simulink model "stableMDS_variable_stiffness"  (R2020b)
settings: Solver=FixedStepAuto  StartTime=0.0  StopTime=10.0  FixedStep=0.001  RelTol=1e-3
values from neighbouring files (symbols this model uses):
  a0 = 0.99    [init.m]
  berta = 0.98    [init.m]
  csi = 1    [init.m]
  e_max = 0.05    [init.m]
  F_max = [2;2]    [init.m]
  F_weight = [0;-50]    [init.m]
  M = 1    [init.m]
  mass = 1    [init.m]
libraries: cstblocks x2
settings Model: Creator=chiara-s  LastModifiedBy=chiara-s

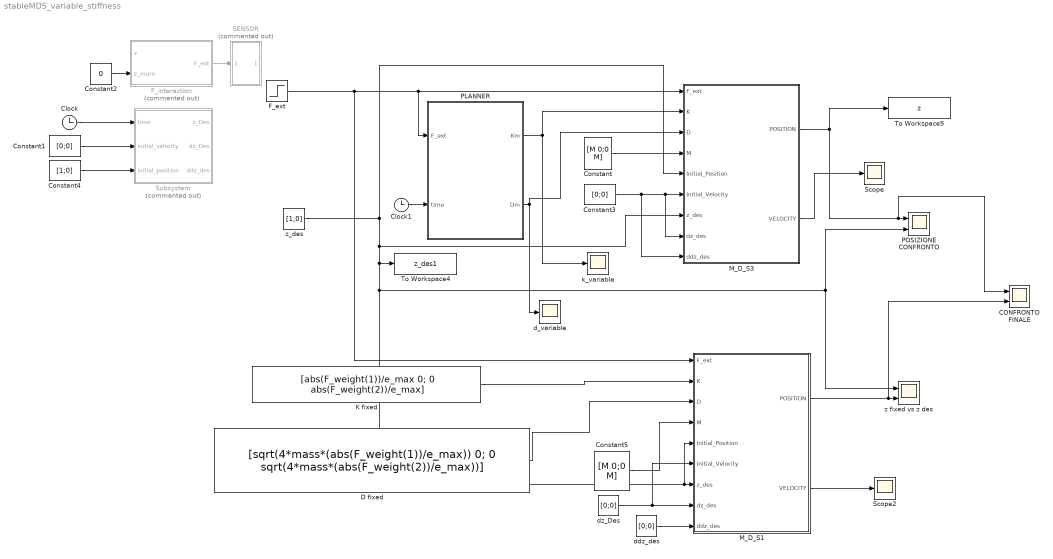
== system stableMDS_variable_stiffness ==
  CONFRONTO FINALE : Scope  NumInputPorts=2
  Clock : Clock
  Clock1 : Clock
  Constant : Constant  Value=[M 0;0 M]
  Constant1 : Constant  Value=[0;0]
  Constant2 : Constant  Value=0
  Constant3 : Constant  Value=[0;0]
  Constant4 : Constant  Value=[1;0]
  Constant5 : Constant  Value=[M 0;0 M]
  D fixed : Constant  Value=[sqrt(4*mass*(abs(F_weight(1))/e_max)) 0; 0 sqrt(4*mass*(abs(F_weight(2))/e_max))]
  F_ext : Step  Before=[0;0]  After=2*F_weight  SampleTime=0
  F_interaction : MATLAB Function  Commented=on  TreatAsAtomicUnit=on
  K fixed : Constant  Value=[abs(F_weight(1))/e_max 0; 0 abs(F_weight(2))/e_max]
  M_D_S1 : Subsystem
  M_D_S3 : Subsystem
  PLANNER : MATLAB Function  TreatAsAtomicUnit=on
  POSIZIONE CONFRONTO : Scope  NumInputPorts=2
  SENSOR : Subsystem  Commented=on
  Scope : Scope
  Scope2 : Scope
  Subsystem : Subsystem  Commented=on
  To Workspace4 : ToWorkspace  VariableName=z_des1  SaveFormat=Structure With Time  SampleTime=-1
      settings: Save2DSignal=2-D array (concatenate along first dimension)
  To Workspace5 : ToWorkspace  VariableName=z  SaveFormat=Structure With Time  SampleTime=-1
  d_variable : Scope
  ddz_des : Constant  Value=[0;0]
  dz_Des : Constant  Value=[0;0]
  k_variable : Scope
  z fixed vs z des : Scope  NumInputPorts=2
  z_des : Constant  Value=[1;0]
  wires:
  M_D_S3/2(VELOCITY) -> Scope/1
  ddz_des/1 -> M_D_S1/9(ddz_des)
  dz_Des/1 -> M_D_S1/8(dz_des), M_D_S1/6(Initial_Velocity)
  Constant4/1 -> Subsystem/3(initial_position)
  Constant1/1 -> Subsystem/2(initial_velocity)
  z_des/1 -> M_D_S3/5(Initial_Position), M_D_S1/5(Initial_Position), M_D_S1/7(z_des), z fixed vs z des/1, POSIZIONE CONFRONTO/2, To Workspace4/1, M_D_S3/7(z_des)
  PLANNER/1(Km) -> k_variable/1, M_D_S3/2(K)
  M_D_S3/1(POSITION) -> To Workspace5/1, CONFRONTO FINALE/1, POSIZIONE CONFRONTO/1
  F_interaction/1(F_ext) -> SENSOR/1(In1)
  Constant2/1 -> F_interaction/2(z_muro)
  D fixed/1 -> M_D_S1/3(D)
  Constant/1 -> M_D_S3/4(M)
  PLANNER/2(Dm) -> M_D_S3/3(D), d_variable/1
  K fixed/1 -> M_D_S1/2(K)
  Clock/1 -> Subsystem/1(time)
  Constant3/1 -> M_D_S3/6(Initial_Velocity), M_D_S3/8(dz_des), M_D_S3/9(ddz_des)
  M_D_S1/2(VELOCITY) -> Scope2/1
  Constant5/1 -> M_D_S1/4(M)
  M_D_S1/1(POSITION) -> CONFRONTO FINALE/2, z fixed vs z des/2
  Clock1/1 -> PLANNER/2(time)
  F_ext/1 -> PLANNER/1(F_ext), M_D_S3/1(F_ext), M_D_S1/1(F_ext)

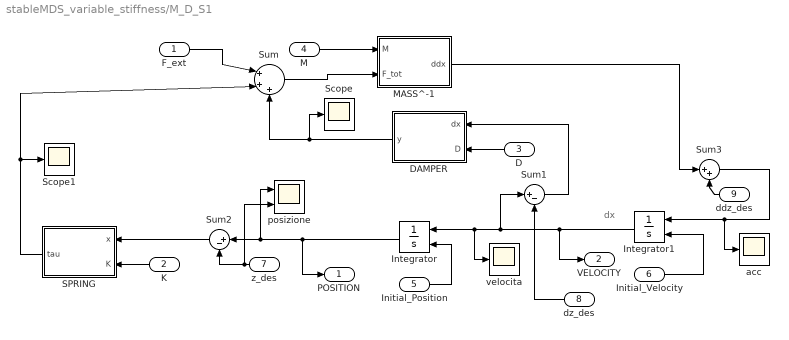
== system stableMDS_variable_stiffness/M_D_S1 ==
  note: dx
  F_ext : Inport
  K : Inport  Port=2
  D : Inport  Port=3
  M : Inport  Port=4
  Initial_Position : Inport  Port=5
  Initial_Velocity : Inport  Port=6
  z_des : Inport  Port=7
  dz_des : Inport  Port=8
  ddz_des : Inport  Port=9
  DAMPER : MATLAB Function  TreatAsAtomicUnit=on
  Integrator : Integrator  InitialConditionSource=external
  Integrator1 : Integrator  InitialConditionSource=external
  MASS^-1 : MATLAB Function  TreatAsAtomicUnit=on
  SPRING : MATLAB Function  TreatAsAtomicUnit=on
  Scope : Scope
  Scope1 : Scope
  Sum : Sum  Inputs=|+++
  Sum1 : Sum  Inputs=|+-
  Sum2 : Sum  Inputs=|+-
  Sum3 : Sum  Inputs=|++
  acc : Scope
  posizione : Scope  NumInputPorts=2
  velocita : Scope
  POSITION : Outport
  VELOCITY : Outport  Port=2
  wires:
  Integrator1/1 -> velocita/1, Integrator/1, Sum1/1, VELOCITY/1
  SPRING/1(tau) -> Sum/2, Scope1/1
  Integrator/1 -> posizione/1, Sum2/1, POSITION/1
  DAMPER/1(y) -> Scope/1, Sum/3
  Sum/1 -> MASS^-1/2(F_tot)
  M/1 -> MASS^-1/1(M)
  D/1 -> DAMPER/2(D)
  K/1 -> SPRING/2(K)
  Initial_Velocity/1 -> Integrator1/2
  Initial_Position/1 -> Integrator/2
  z_des/1 -> posizione/2, Sum2/2
  Sum2/1 -> SPRING/1(x)
  MASS^-1/1(ddx) -> Sum3/1
  Sum1/1 -> DAMPER/1(dx)
  Sum3/1 -> acc/1, Integrator1/1
  dz_des/1 -> Sum1/2
  ddz_des/1 -> Sum3/2
  F_ext/1 -> Sum/1

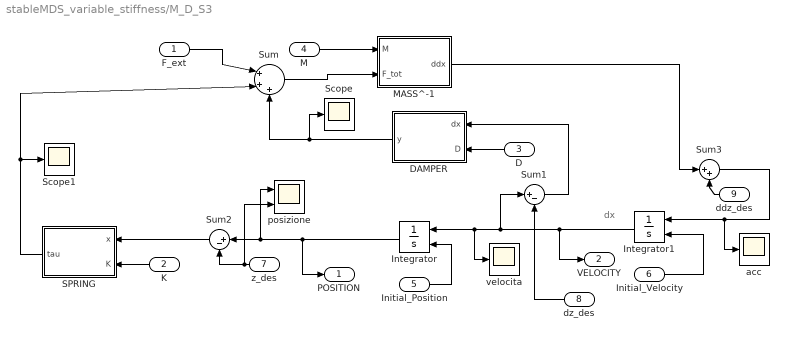
== system stableMDS_variable_stiffness/M_D_S3 ==
  note: dx
  F_ext : Inport
  K : Inport  Port=2
  D : Inport  Port=3
  M : Inport  Port=4
  Initial_Position : Inport  Port=5
  Initial_Velocity : Inport  Port=6
  z_des : Inport  Port=7
  dz_des : Inport  Port=8
  ddz_des : Inport  Port=9
  DAMPER : MATLAB Function  TreatAsAtomicUnit=on
  Integrator : Integrator  InitialConditionSource=external
  Integrator1 : Integrator  InitialConditionSource=external
  MASS^-1 : MATLAB Function  TreatAsAtomicUnit=on
  SPRING : MATLAB Function  TreatAsAtomicUnit=on
  Scope : Scope
  Scope1 : Scope
  Sum : Sum  Inputs=|+++
  Sum1 : Sum  Inputs=|+-
  Sum2 : Sum  Inputs=|+-
  Sum3 : Sum  Inputs=|++
  acc : Scope
  posizione : Scope  NumInputPorts=2
  velocita : Scope
  POSITION : Outport
  VELOCITY : Outport  Port=2
  wires:
  Integrator1/1 -> velocita/1, Integrator/1, Sum1/1, VELOCITY/1
  SPRING/1(tau) -> Sum/2, Scope1/1
  Integrator/1 -> posizione/1, Sum2/1, POSITION/1
  DAMPER/1(y) -> Scope/1, Sum/3
  Sum/1 -> MASS^-1/2(F_tot)
  M/1 -> MASS^-1/1(M)
  D/1 -> DAMPER/2(D)
  K/1 -> SPRING/2(K)
  Initial_Velocity/1 -> Integrator1/2
  Initial_Position/1 -> Integrator/2
  z_des/1 -> posizione/2, Sum2/2
  Sum2/1 -> SPRING/1(x)
  MASS^-1/1(ddx) -> Sum3/1
  Sum1/1 -> DAMPER/1(dx)
  Sum3/1 -> acc/1, Integrator1/1
  dz_des/1 -> Sum1/2
  ddz_des/1 -> Sum3/2
  F_ext/1 -> Sum/1

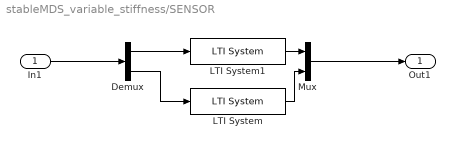
== system stableMDS_variable_stiffness/SENSOR ==
  In1 : Inport
  Demux : Demux  Outputs=2
  LTI System : cstblocks/LTI System  sys=tf(200^2,[1 0.5*2*200 200^2])  IC=[]
  LTI System1 : cstblocks/LTI System  sys=tf(200^2,[1 0.5*2*200 200^2])  IC=[]
  Mux : Mux  Inputs=2
  Out1 : Outport
  wires:
  LTI System1/1 -> Mux/1
  Demux/1 -> LTI System1/1
  Demux/2 -> LTI System/1
  LTI System/1 -> Mux/2
  Mux/1 -> Out1/1
  In1/1 -> Demux/1

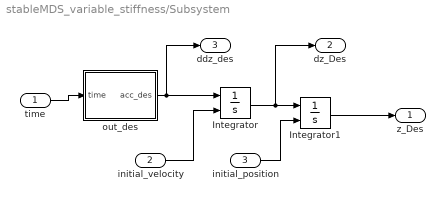
== system stableMDS_variable_stiffness/Subsystem ==
  time : Inport
  initial_velocity : Inport  Port=2
  initial_position : Inport  Port=3
  Integrator : Integrator  InitialConditionSource=external
  Integrator1 : Integrator  InitialConditionSource=external
  out_des : MATLAB Function  TreatAsAtomicUnit=on
  z_Des : Outport
  dz_Des : Outport  Port=2
  ddz_des : Outport  Port=3
  wires:
  Integrator1/1 -> z_Des/1
  time/1 -> out_des/1(time)
  Integrator/1 -> dz_Des/1, Integrator1/1
  out_des/1(acc_des) -> ddz_des/1, Integrator/1
  initial_velocity/1 -> Integrator/2
  initial_position/1 -> Integrator1/2

== matlab function stableMDS_variable_stiffness/Subsystem/out_des ==
  settings: sampleTime=0.1
  data: time input; acc_des output
function acc_des = fcn(time)
%% desired trajectory generator
if time < 0.1
    acc_des = [-5;0]; 
elseif time < 3.1
    acc_des = [0;0];
elseif time < 3.2
    acc_des = [5;0];
else 
    acc_des = [0;0];
end


end

== matlab function stableMDS_variable_stiffness/F_interaction ==
  data: z input; F_ext output; z_muro input
function F_ext = fcn(z, z_muro)
% hypothesis: table reaction force with elastic behaviour
F_ext = zeros(2,1);
K = 10000;         % 1 mm displacement for 10 kg
F_ext(1) = 0;
F_ext(2) = 0;
% if contact is happened
if z_muro > z(1)
    F_ext(1) = K*(z_muro - z(1));
end

== matlab function stableMDS_variable_stiffness/M_D_S1/DAMPER ==
  data: dx input; y output; D input
function y = fcn(dx, D)
y = - D*dx;
end

== matlab function stableMDS_variable_stiffness/M_D_S1/MASS^-1 ==
  data: M input; ddx output; F_tot input
function ddx = fcn(M,F_tot)
ddx = (M^-1)*F_tot;
end

== matlab function stableMDS_variable_stiffness/M_D_S1/SPRING ==
  data: x input; tau output; K input
function tau = fcn(x, K)
tau= -K*x;
end

== matlab function stableMDS_variable_stiffness/M_D_S3/DAMPER ==
  data: dx input; y output; D input
function y = fcn(dx, D)
y = - D*dx;
end

== matlab function stableMDS_variable_stiffness/M_D_S3/MASS^-1 ==
  data: M input; ddx output; F_tot input
function ddx = fcn(M,F_tot)
ddx = (M^-1)*F_tot;
end

== matlab function stableMDS_variable_stiffness/M_D_S3/SPRING ==
  data: x input; tau output; K input
function tau = fcn(x, K)
tau= -K*x;
end

== matlab function stableMDS_variable_stiffness/PLANNER ==
  settings: updateMethod=DISCRETE
  data: Km output; Dm output; e_max parameter; F_max parameter; F_ext input; mass parameter; F_weight parameter; time input; a0 parameter; csi parameter; berta parameter
function [Km,Dm] = fcn(e_max, F_max, F_ext, mass, F_weight, time, a0, csi, berta)

% with an estimated weight, k and d increase 
%% Outputs
% Km            stiffness matrix
% Dm            damping matrix 
%% Inputs
% time          current simulation time
% F_ext         measured external force

% variables initialization 
persistent kx_i ky_i dx dy timeG kx ky F_grasp kx_f ky_f

if isempty(kx_f)
    kx_f = abs(F_weight(1))/e_max;
end

if isempty(ky_f)
    ky_f = abs(F_weight(2))/e_max;
end

if isempty(F_grasp)
    F_grasp = [0;0];
end

if isempty(timeG)
    timeG = 1000;
end

if isempty(kx)
   kx = abs(F_weight(1))/e_max; 
end
if isempty(ky)
   ky = abs(F_weight(2))/e_max;
end

% initialization of k and d 
if isempty(kx_i)
   kx_i = abs(F_weight(1))/e_max; 
end
if isempty(ky_i)
   ky_i = abs(F_weight(2))/e_max;
end
if isempty(dx)
    dx = sqrt(4*kx_i*mass);
end
if isempty(dy)
    dy = sqrt(4*ky_i*mass);
end

% definition of k_dot for stability condition (from article)
k_dotx = berta*(4*a0*sqrt(kx_i/mass)*(kx_i)^(3/2))/(sqrt(kx_i) + 2*a0*csi*sqrt(kx_i));
k_doty = berta*(4*a0*sqrt(ky_i/mass)*(ky_i)^(3/2))/(sqrt(ky_i) + 2*a0*csi*sqrt(ky_i));


% start algoritm with k variable
if abs(F_ext(1))/kx > e_max
    if timeG == 1000
        timeG = time;
    end
    kx_f = abs(F_ext(1))/e_max;
    % law for increasing k
    k_tempx = kx_i + k_dotx*(time -timeG);
    if k_tempx > kx_f
        kx = kx_f;
    else
        kx = k_tempx;
    end
    dx = sqrt(4*kx*mass);
    
end
if abs(F_ext(2))/ky > e_max
    if timeG == 1000
        timeG = time;
    end
    ky_f = abs(F_ext(2))/e_max;
    k_tempy = ky_i + k_doty*(time -timeG);
    if k_tempy > ky_f
        ky = ky_f;
    else
        ky = k_tempy;
    end
    dy = sqrt(4*ky*mass);
end

% set k istantaneously
% kx = abs(F_ext(1))/e_max;
% ky = abs(F_ext(2))/e_max;

% Final Values of D-K
Dm = diag([dx,dy]);
Km = diag([kx,ky]);

end
